simulink model "prbs_8bits"  (Simulink 6.6)
settings: Solver=FixedStepDiscrete  StartTime=0.0  StopTime=255  FixedStep=1  RelTol=1e-3
undefined symbols (not defined in the file): TS_PRBS
settings Model: Creator=bailly  LastModifiedBy=bailly

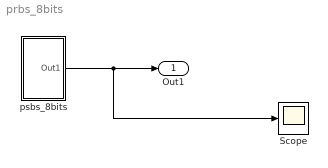
== system prbs_8bits ==
  Scope : Scope
  psbs_8bits : Subsystem
  Out1 : Outport
  wires:
  psbs_8bits/1(Out1) -> Out1/1, Scope/1

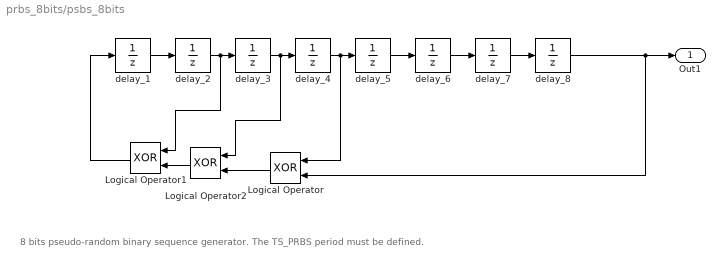
== system prbs_8bits/psbs_8bits ==
  note: 8 bits pseudo-random binary sequence generator.
      | The TS_PRBS period must be defined.
  Logical Operator : Logic  Orientation=left  Operator=XOR  AllPortsSameDT=off  OutDataTypeMode=Boolean
  Logical Operator1 : Logic  Orientation=left  Operator=XOR  AllPortsSameDT=off  OutDataTypeMode=Boolean
  Logical Operator2 : Logic  Orientation=left  Operator=XOR  AllPortsSameDT=off  OutDataTypeMode=Boolean
  delay_1 : UnitDelay  X0=TS_PRBS  SampleTime=-1
  delay_{2..8} (7 alike) : UnitDelay  X0=1  SampleTime=-1
  Out1 : Outport
  wires:
  delay_5/1 -> delay_6/1
  delay_6/1 -> delay_7/1
  delay_2/1 -> delay_3/1, Logical Operator1/1
  delay_3/1 -> delay_4/1, Logical Operator2/1
  delay_4/1 -> delay_5/1, Logical Operator/1
  delay_1/1 -> delay_2/1
  delay_7/1 -> delay_8/1
  delay_8/1 -> Logical Operator/2, Out1/1
  Logical Operator1/1 -> delay_1/1
  Logical Operator2/1 -> Logical Operator1/2
  Logical Operator/1 -> Logical Operator2/2
